simulink model "cascadingblock_referenced"  (R2020b)
settings: Solver=FixedStepDiscrete  StartTime=0.0  StopTime=1  FixedStep=0.01  RelTol=1e-3
settings Model: Creator=abhin  LastModifiedBy=abhin
settings DataIOCC: SaveOutput=off  SaveTime=off

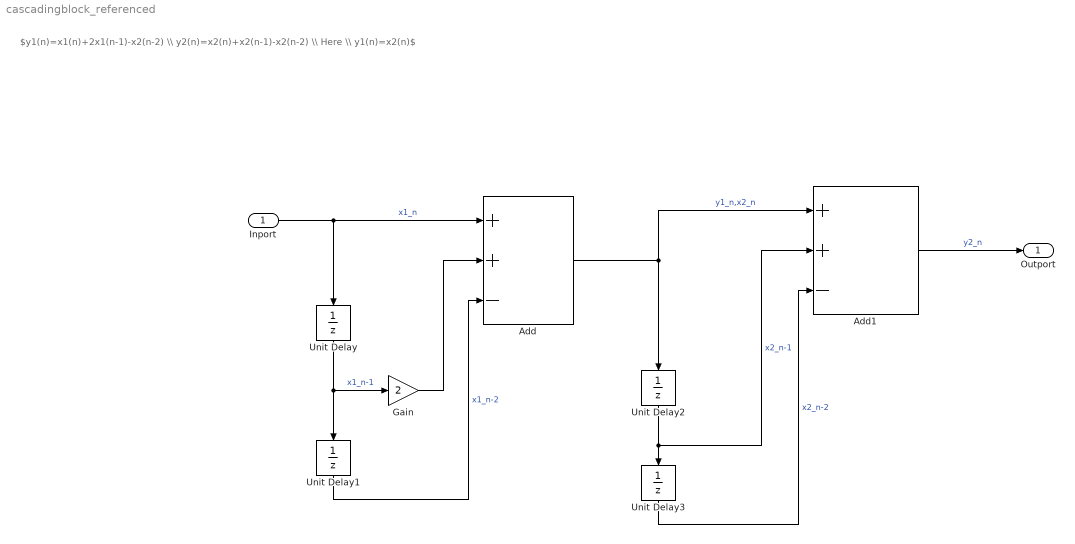
== system cascadingblock_referenced ==
  note: $y1(n)=x1(n)+2x1(n-1)-x2(n-2) \\ y2(n)=x2(n)+x2(n-1)-x2(n-2) \\ Here \\ y1(n)=x2(n)$
  Inport : Inport  OutDataTypeStr=double  PortDimensions=1  SampleTime=[0.01,0]
  Add : Sum  Inputs=++-
  Add1 : Sum  Inputs=++-
  Gain : Gain  Gain=2
  Unit Delay{,1..3} (4 alike) : UnitDelay  SampleTime=-1  HasFrameUpgradeWarning=on
  Outport : Outport  OutDataTypeStr=double  PortDimensions=1  SampleTime=[0.01,0]
  wires:
  Add1/1 -> Outport/1  "y2_n"
  Unit Delay/1 -> Gain/1, Unit Delay1/1  "x1_n-1"
  Add/1 -> Add1/1, Unit Delay2/1  "y1_n,x2_n"
  Inport/1 -> Unit Delay/1, Add/1  "x1_n"
  Unit Delay2/1 -> Unit Delay3/1, Add1/2  "x2_n-1"
  Gain/1 -> Add/2
  Unit Delay1/1 -> Add/3  "x1_n-2"
  Unit Delay3/1 -> Add1/3  "x2_n-2"
